simulink model "PENDULO_CARRO_NO_LINEAL2"  (R2018a)
settings: Solver=VariableStepAuto  StartTime=0.0  StopTime=10.0  RelTol=1e-3
values from neighbouring files (symbols this model uses):
  g = 9.81    [ParametrosPenduloInvertido.m]
  l = 0.45    [ParametrosPenduloInvertido.m]
  M = 2    [ParametrosPenduloInvertido.m]
  m = 0.5    [ParametrosPenduloInvertido.m]
undefined symbols (not defined in the file or in its folder): b1
libraries: fuzblock x1
settings Model: Creator=Omie-PC  LastModifiedBy=Omie-PC

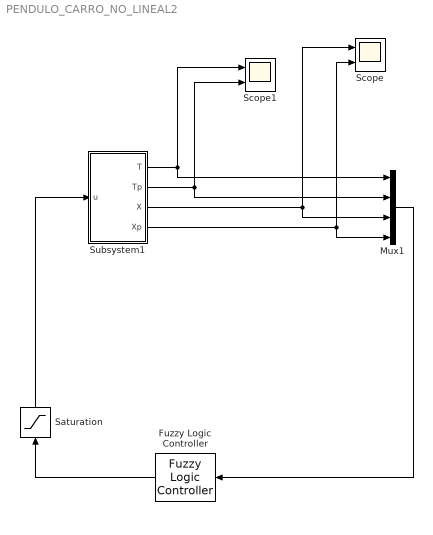
== system PENDULO_CARRO_NO_LINEAL2 ==
  Fuzzy Logic Controller : fuzblock/Fuzzy Logic  Controller  FIS=TS_carro_pendulo  OutputSampleNumber=101  DataType=double  FuzzifiedInputs=off  RuleFiringStrengths=off  RuleOutputs=off  AggregatedOutputs=off  SimulateUsing=Interpreted execution  OutOfRangeInputValueMessage=warning  NoRuleFiredMessage=warning  EmptyOutputFuzzySetMessage=warning
  Mux1 : Mux
  Saturation : Saturate  UpperLimit=7  LowerLimit=-7
  Scope : Scope  NumInputPorts=2
  Scope1 : Scope  NumInputPorts=2
  Subsystem1 : Subsystem
  wires:
  Fuzzy Logic Controller/1 -> Saturation/1
  Saturation/1 -> Subsystem1/1(u)
  Subsystem1/1(T) -> Scope1/1, Mux1/1
  Subsystem1/2(Tp) -> Scope1/2, Mux1/2
  Subsystem1/3(X) -> Scope/1, Mux1/3
  Subsystem1/4(Xp) -> Mux1/4, Scope/2
  Mux1/1 -> Fuzzy Logic Controller/1

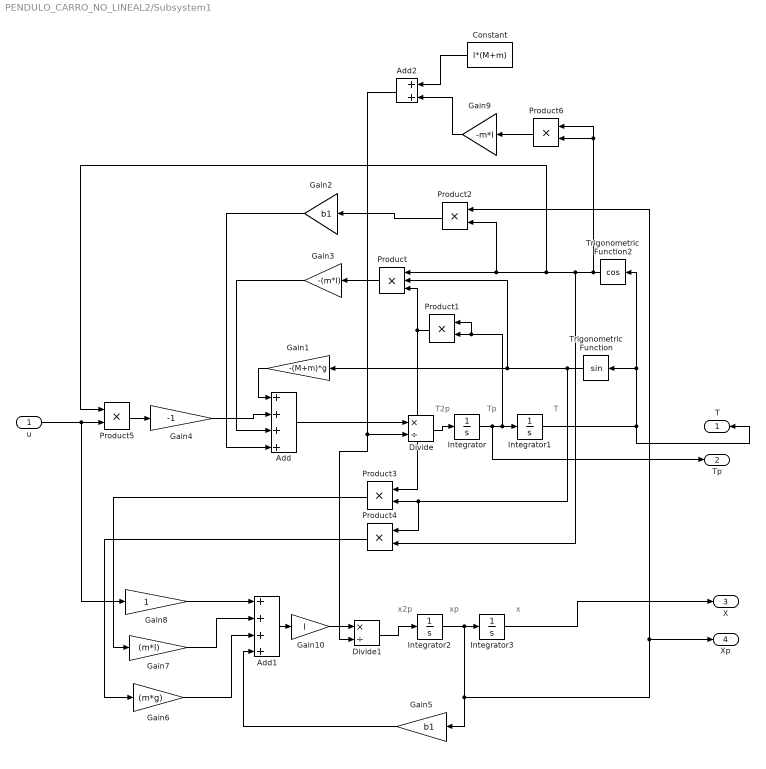
== system PENDULO_CARRO_NO_LINEAL2/Subsystem1 ==
  note: Tp
  note: T2p
  note: T
  note: x
  note: xp
  note: x2p
  u : Inport
  Add : Sum  Inputs=++++
  Add1 : Sum  Inputs=++++
  Add2 : Sum
  Constant : Constant  Value=l*(M+m)
  Divide : Product  Inputs=*/
  Divide1 : Product  Inputs=*/
  Gain1 : Gain  Gain=-(M+m)*g
  Gain10 : Gain  Gain=l
  Gain2 : Gain  Gain=b1
  Gain3 : Gain  Gain=-(m*l)
  Gain4 : Gain  Gain=-1
  Gain5 : Gain  Gain=b1
  Gain6 : Gain  Gain=(m*g)
  Gain7 : Gain  Gain=(m*l)
  Gain8 : Gain
  Gain9 : Gain  Gain=-m*l
  Integrator : Integrator
  Integrator1 : Integrator  InitialCondition=pi
  Integrator2 : Integrator  InitialCondition=0.1
  Integrator3 : Integrator
  Product : Product  Inputs=3
  Product{1..6} (6 alike) : Product
  Trigonometric Function : Trigonometry
  Trigonometric Function2 : Trigonometry  Operator=cos
  T : Outport
  Tp : Outport  Port=2
  X : Outport  Port=3
  Xp : Outport  Port=4
  wires:
  u/1 -> Product5/2, Gain8/1
  Product5/1 -> Gain4/1
  Integrator1/1 -> T/1, Trigonometric Function2/1, Trigonometric Function/1
  Trigonometric Function/1 -> Product4/1, Product3/2, Gain1/1, Product/2
  Gain4/1 -> Add/2
  Product1/1 -> Product3/1, Product/3
  Integrator/1 -> Integrator1/1, Product1/1, Product1/2, Tp/1
  Product2/1 -> Gain2/1
  Product4/1 -> Gain6/1
  Gain1/1 -> Add/1
  Gain6/1 -> Add1/3
  Gain8/1 -> Add1/1
  Gain7/1 -> Add1/2
  Product3/1 -> Gain7/1
  Gain2/1 -> Add/4
  Integrator2/1 -> Xp/1, Product2/1, Gain5/1, Integrator3/1
  Gain3/1 -> Add/3
  Gain5/1 -> Add1/4
  Product/1 -> Gain3/1
  Integrator3/1 -> X/1
  Divide/1 -> Integrator/1
  Trigonometric Function2/1 -> Product6/1, Product6/2, Product4/2, Product2/2, Product/1, Product5/1
  Add/1 -> Divide/1
  Divide1/1 -> Integrator2/1
  Gain9/1 -> Add2/2
  Constant/1 -> Add2/1
  Product6/1 -> Gain9/1
  Add2/1 -> Divide1/2, Divide/2
  Add1/1 -> Gain10/1
  Gain10/1 -> Divide1/1
